simulink model "boost_CM_switching"  (Simulink 6.5)
settings: Solver=ode45  StartTime=0.0  StopTime=1000e-6  MaxStep=0.1e-6  RelTol=1e-3
settings Model: Creator=Mama  LastModifiedBy=Dragan Maksimovic
settings DebuggingCC: AlgebraicLoopMsg=none  SolverPrmCheckMsg=none  UnconnectedOutputMsg=none

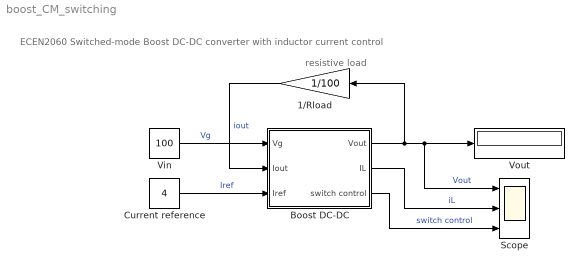
== system boost_CM_switching ==
  note: ECEN2060
      | Switched-mode Boost
      | DC-DC converter
      | with inductor current control
  note: resistive load
  1/Rload : Gain  Orientation=left  Gain=1/100
  Boost DC-DC : Subsystem  mask{L=200e-6, DeltaI=1, C=10e-6, Vo=200}
      mask prompts: L "Inductance"; DeltaI "Inductor current ripple"; C "Capacitance"; Vo "Initial capacitor voltage"
      mask help: Switched-mode Boost (step-up) DC-DC converter (switching). Inductor current, which is the input current of the converter, is controlled by a comparator with hysteresis. The model is ideal, losses are neglected, efficiency is 100%
      mask Display:
      | text(0.5,0.8,'Boost','horizontalAlignment', 'center');
      | text(0.5,0.65,'DC-DC','horizontalAlignment', 'center');
      | text(0.5,0.5,'(switching)','horizontalAlignment', 'center');
      | text(0.5,0.35,'current control','horizontalAlignment', 'center');
  Current reference : Constant  Value=4  OutDataType=sfix(16)  ConRadixGroup=Use specified scaling  OutScaling=2^0  SampleTime=inf  FramePeriod=inf
  Scope : Scope  NumInputPorts=3
      settings: TimeRange=0.001  YMin=198~0~0  YMax=200~6~1
  Vin : Constant  Value=100  OutDataType=sfix(16)  ConRadixGroup=Use specified scaling  OutScaling=2^0  SampleTime=inf  FramePeriod=inf
  Vout : Display
  wires:
  Current reference/1 -> Boost DC-DC/3(Iref)  "Iref"
  Vin/1 -> Boost DC-DC/1(Vg)  "Vg"
  Boost DC-DC/1(Vout) -> Vout/1, Scope/1, 1/Rload/1  "Vout"
  Boost DC-DC/2(IL) -> Scope/2  "iL"
  Boost DC-DC/3(switch control) -> Scope/3  "switch control"
  1/Rload/1 -> Boost DC-DC/2(Iout)  "iout"

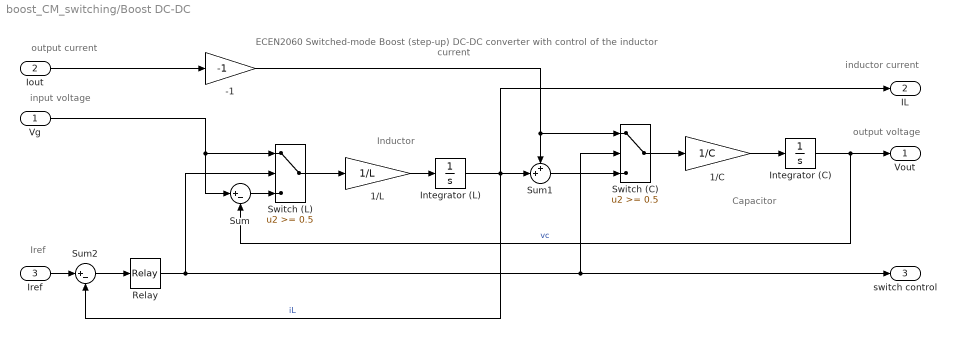
== system boost_CM_switching/Boost DC-DC ==
  note: ECEN2060 Switched-mode Boost (step-up) DC-DC converter
      | with control of the inductor current
  note: output voltage
  note: inductor current
  note: output current
  note: input voltage
  note: Iref
  note: Inductor
  note: Capacitor
  Vg : Inport
  Iout : Inport  Port=2
  Iref : Inport  Port=3
  -1 : Gain  Gain=-1
  1/C : Gain  Gain=1/C
  1/L : Gain  Gain=1/L
  Integrator (C) : Integrator  InitialCondition=Vo
  Integrator (L) : Integrator
  Relay : Relay  OnSwitchValue=DeltaI/2  OffSwitchValue=-DeltaI/2
  Sum : Sum  Inputs=|+-
  Sum1 : Sum  Inputs=++|
  Sum2 : Sum  Inputs=|+-
  Switch (C) : Switch  Threshold=0.5
  Switch (L) : Switch  Threshold=0.5
  Vout : Outport
  IL : Outport  Port=2
  switch control : Outport  Port=3
  wires:
  Vg/1 -> Switch (L)/1, Sum/1
  Relay/1 -> Switch (L)/2, Switch (C)/2, switch control/1
  Sum/1 -> Switch (L)/3
  Sum1/1 -> Switch (C)/3
  Switch (C)/1 -> 1/C/1
  1/C/1 -> Integrator (C)/1
  Integrator (C)/1 -> Sum/2, Vout/1  "vc"
  Switch (L)/1 -> 1/L/1
  1/L/1 -> Integrator (L)/1
  Integrator (L)/1 -> Sum1/2, IL/1, Sum2/2  "iL"
  Iref/1 -> Sum2/1
  Iout/1 -> -1/1
  -1/1 -> Sum1/1, Switch (C)/1
  Sum2/1 -> Relay/1
